simulink model "SistemaP4"  (R2024b)
settings: Solver=ode15s  StartTime=0.0  StopTime=10  RelTol=1e-3
settings DataIOCC: SaveOutput=off  SignalLogging=off  DSMLogging=off  SaveTime=off  ReturnWorkspaceOutputs=off

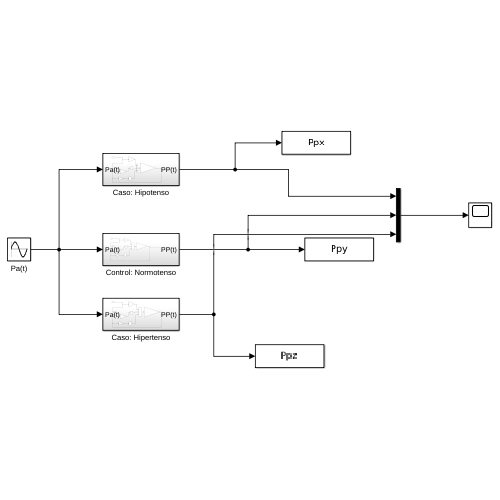
[thumbnail: Simulink's stored preview of the top-level diagram]
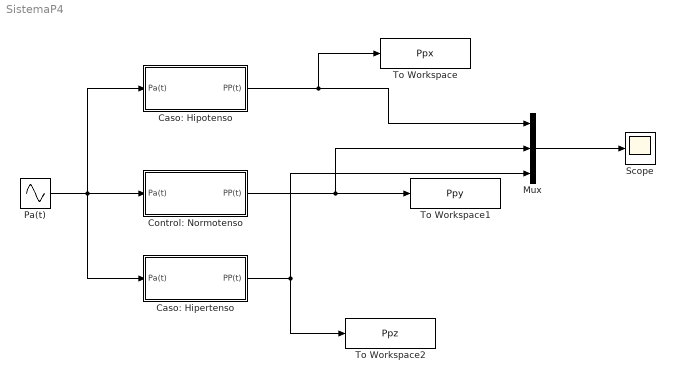
== system SistemaP4 ==
  Caso: Hipertenso : Subsystem
  Caso: Hipotenso : Subsystem
  Control: Normotenso : Subsystem
  Mux : Mux  Inputs=3
  Pa(t) : Sin  Frequency=2*pi*(95/61)  SampleTime=0
  Scope : Scope
  To Workspace : ToWorkspace  VariableName=Ppx  SaveFormat=Timeseries  SampleTime=-1
  To Workspace1 : ToWorkspace  VariableName=Ppy  SaveFormat=Timeseries  SampleTime=-1
  To Workspace2 : ToWorkspace  VariableName=Ppz  SaveFormat=Timeseries  SampleTime=-1
  wires:
  Mux/1 -> Scope/1
  Pa(t)/1 -> Caso: Hipertenso/1(Pa(t)), Control: Normotenso/1(Pa(t)), Caso: Hipotenso/1(Pa(t))
  Control: Normotenso/1(PP(t)) -> Mux/2, To Workspace1/1
  Caso: Hipotenso/1(PP(t)) -> To Workspace/1, Mux/1
  Caso: Hipertenso/1(PP(t)) -> To Workspace2/1, Mux/3

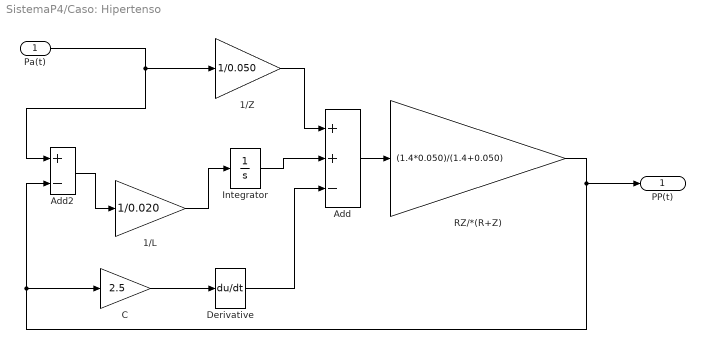
== system SistemaP4/Caso: Hipertenso ==
  Pa(t) : Inport
  1/L : Gain  Gain=1/0.020
  1/Z : Gain  Gain=1/0.050
  Add : Sum  Inputs=++-
  Add2 : Sum  Inputs=+-
  C : Gain  Gain=2.5
  Derivative : Derivative
  Integrator : Integrator
  RZ/*(R+Z) : Gain  Gain=(1.4*0.050)/(1.4+0.050)
  PP(t) : Outport
  wires:
  Add/1 -> RZ/*(R+Z)/1
  Pa(t)/1 -> Add2/1, 1/Z/1
  Derivative/1 -> Add/3
  RZ/*(R+Z)/1 -> C/1, Add2/2, PP(t)/1
  C/1 -> Derivative/1
  1/L/1 -> Integrator/1
  Add2/1 -> 1/L/1
  Integrator/1 -> Add/2
  1/Z/1 -> Add/1

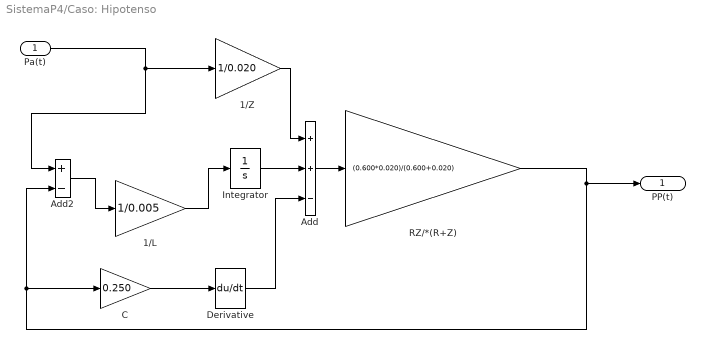
== system SistemaP4/Caso: Hipotenso ==
  Pa(t) : Inport
  1/L : Gain  Gain=1/0.005
  1/Z : Gain  Gain=1/0.020
  Add : Sum  Inputs=++-
  Add2 : Sum  Inputs=+-
  C : Gain  Gain=0.250
  Derivative : Derivative
  Integrator : Integrator
  RZ/*(R+Z) : Gain  Gain=(0.600*0.020)/(0.600+0.020)
  PP(t) : Outport
  wires:
  1/L/1 -> Integrator/1
  C/1 -> Derivative/1
  Integrator/1 -> Add/2
  Derivative/1 -> Add/3
  Add2/1 -> 1/L/1
  Add/1 -> RZ/*(R+Z)/1
  Pa(t)/1 -> Add2/1, 1/Z/1
  RZ/*(R+Z)/1 -> C/1, Add2/2, PP(t)/1
  1/Z/1 -> Add/1

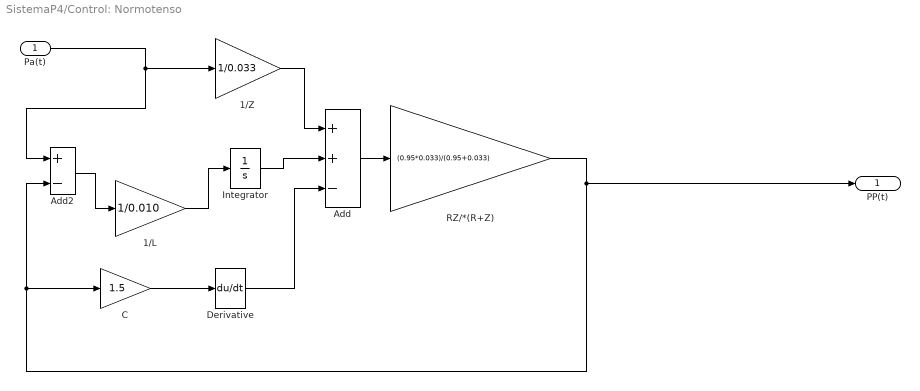
== system SistemaP4/Control: Normotenso ==
  Pa(t) : Inport
  1/L : Gain  Gain=1/0.010
  1/Z : Gain  Gain=1/0.033
  Add : Sum  Inputs=++-
  Add2 : Sum  Inputs=+-
  C : Gain  Gain=1.5
  Derivative : Derivative
  Integrator : Integrator
  RZ/*(R+Z) : Gain  Gain=(0.95*0.033)/(0.95+0.033)
  PP(t) : Outport
  wires:
  1/L/1 -> Integrator/1
  C/1 -> Derivative/1
  1/Z/1 -> Add/1
  Derivative/1 -> Add/3
  Add/1 -> RZ/*(R+Z)/1
  Add2/1 -> 1/L/1
  RZ/*(R+Z)/1 -> C/1, Add2/2, PP(t)/1
  Pa(t)/1 -> Add2/1, 1/Z/1
  Integrator/1 -> Add/2
